simulink model "Sum6"  (R2017b)
settings: Solver=FixedStepDiscrete  StartTime=0.0  StopTime=10.0  FixedStep=0.200000  RelTol=1e-3
settings Model: Creator=hbourbou  LastModifiedBy=hbourbou
settings DataIOCC: SaveFormat=StructureWithTime
settings OptimizationCC: LifeSpan=inf
settings DebuggingCC: SFExecutionAtInitializationDiag=none
settings HardwareCC: ProdBitPerSizeT=32  ProdBitPerPtrDiffT=32  ProdWordSize=32  ProdHWDeviceType=Specified
settings CodeAppCC: StateflowObjectComments=on

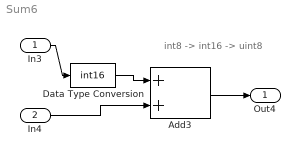
== system Sum6 ==
  note: int8 -> int16 -> uint8
  In3 : Inport  OutDataTypeStr=int8
  In4 : Inport  Port=2  OutDataTypeStr=int16
  Add3 : Sum
  Data Type Conversion : DataTypeConversion  OutDataTypeStr=int16
  Out4 : Outport
  wires:
  Add3/1 -> Out4/1
  In3/1 -> Data Type Conversion/1
  In4/1 -> Add3/2
  Data Type Conversion/1 -> Add3/1
